simulink model "CubliMasterModel_Corner"  (R2025b)
settings: Solver=FixedStepAuto  StartTime=0.0  StopTime=10  FixedStep=0.001  RelTol=1e-3
values from neighbouring files (symbols this model uses):
  B0 = atan(-1/sqrt(2))    [CubeMasterModel_Corner.m]
  g = 9.81    [CubeMasterModel_Corner.m]
  IMU_st = 0.005    [CubeMasterModel_Corner.m]
  J_acctuator = J_rw+J_motor    (= 0.000472174)    [CubeMasterModel_Corner.m]
  K = zeros(3,8)    [CubeMasterModel_Corner.m]
  Km = 0.05    [CubeMasterModel_Corner.m]
  KV = 195    [CubeMasterModel_Corner.m]
  m = 3    [CubeMasterModel_Corner.m]
  M_battery = 100    [CubeMasterModel_Corner.m]
  M_core = 70    [CubeMasterModel_Corner.m]
  M_frame = 6*6 + 2.5*4    (= 46)    [CubeMasterModel_Corner.m]
  M_motor = 110    [CubeMasterModel_Corner.m]
  M_PCB = 106.6    [CubeMasterModel_Corner.m]
  M_wheel = 145    [CubeMasterModel_Corner.m]
  T = zeros(9)    [CubeMasterModel_Corner.m]
  Tmax = 0.25    [CubeMasterModel_Corner.m]
  TorqueRate = 0.1/0.005    (= 20)    [CubeMasterModel_Corner.m]
  Ts = 0.005    [CubeMasterModel_Corner.m]
  Y0 = pi/4    (= 0.785398163397)    [CubeMasterModel_Corner.m]
undefined symbols (not defined in the file or in its folder): X, Y, Z
libraries: sm_lib x39, nesl_utility x23, simulink x11
settings Model: Creator=Daniel  LastModifiedBy=Daniel

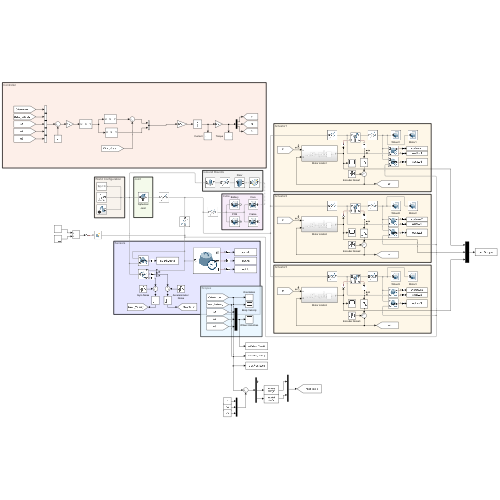
[thumbnail: Simulink's stored preview of the top-level diagram]
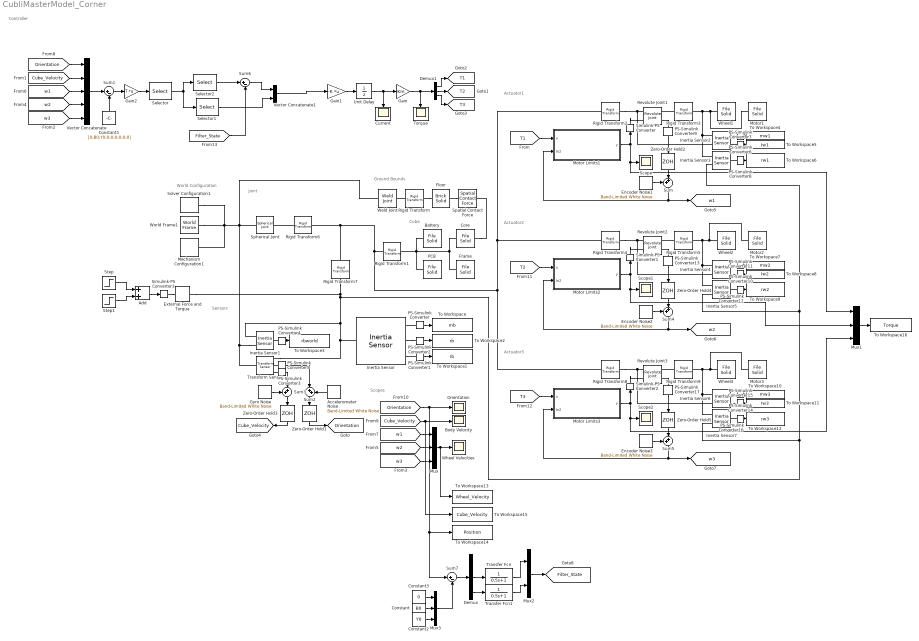
== system CubliMasterModel_Corner ==
  note: Actuator1
  note: Scopes
  note: Sensors
  note: Joint
  note: Cube
  note: Ground Bounds
  note: Controller
  note: World Configuration
  note: Actuator2
  note: Actuator3
  Accelerometer Noise : simulink/Sources/Band-Limited White Noise  Cov=IMU_acc_np  Ts=IMU_st  seed=[23341]
  Add : Sum
  Battery : sm_lib/Body Elements/File Solid  ExtGeomFileName=C:\Users\Daniel\OneDrive - University of Warwick\Documents\MATLAB\Report_Models\Edge Balance\Discretised\BatteryModel.step  UnitType=Custom  ExtGeomFileUnits=mm  StepReaderType=HEX  ExportConvexHullGeometry=on  InertiaType=CalculateFromGeometry  BasedOnType=Mass  Density=1150  DensityUnits=kg/m^3  Mass=M_battery  MassUnits=g  CenterOfMass=COM_battery  CenterOfMassUnits=mm  MomentsOfInertia=I_battery  MomentsOfInertiaUnits=g*mm^2  ProductsOfInertia=P_battery  ProductsOfInertiaUnits=g*mm^2  GraphicType=FromGeometry  MarkerShape=Sphere  MarkerSize=10  GraphicVisPropType=SimpleVisualProperties  GraphicDiffuseColor=[0 0.3 0.1]  GraphicOpacity=1  GraphicSpecularColor=[0.5 0.5 0.5 1.0]  GraphicAmbientColor=[0.15 0.15 0.15 1.0]  GraphicEmissiveColor=[0.0 0.0 0.0 1.0]  GraphicShininess=75  DoExposeReferenceFrame=on  SerializedFrames=<Frames/>
  Body Velocity : Scope
      settings: ActiveDisplayYMinimum=-1224.4716207525835  ActiveDisplayYMaximum=1175.2559397382945  DataLoggingVariableName=ScopeData2
  Constant : Constant  Value=B0
  Constant1 : Constant  Value=[0;B0;Y0;0;0;0;0;0;0]
  Constant2 : Constant  Value=Y0
  Constant3 : Constant  Value=0
  Core : sm_lib/Body Elements/File Solid  ExtGeomFileName=C:\Users\Daniel\OneDrive - University of Warwick\Documents\MATLAB\Report_Models\Edge Balance\Discretised\coreModel.3mf  UnitType=Custom  ExtGeomFileUnits=mm  StepReaderType=HEX  ExportConvexHullGeometry=on  InertiaType=PointMass  BasedOnType=Mass  Density=1150  DensityUnits=kg/m^3  Mass=M_core  MassUnits=g  CenterOfMass=COM_core  CenterOfMassUnits=mm  MomentsOfInertia=I_core  MomentsOfInertiaUnits=g*mm^2  ProductsOfInertia=P_core  ProductsOfInertiaUnits=g*mm^2  GraphicType=FromGeometry  MarkerShape=Sphere  MarkerSize=10  GraphicVisPropType=SimpleVisualProperties  GraphicDiffuseColor=[0.3 0.3 0.3]  GraphicOpacity=1  GraphicSpecularColor=[0.5 0.5 0.5 1.0]  GraphicAmbientColor=[0.15 0.15 0.15 1.0]  GraphicEmissiveColor=[0.0 0.0 0.0 1.0]  GraphicShininess=75  DoExposeReferenceFrame=on  SerializedFrames=<Frames/>
  Current : Scope
      settings: ActiveDisplayYMinimum=-5.2720631408521568  ActiveDisplayYMaximum=8.6725422679254329  DataLoggingVariableName=ScopeData3
  Demux : Demux  Outputs=3
  Demux1 : Demux  Outputs=3
  Encoder Noise1 : simulink/Sources/Band-Limited White Noise  Cov=0  Ts=0.001  seed=[23341]
  Encoder Noise2 : simulink/Sources/Band-Limited White Noise  Cov=0  Ts=0.001  seed=[23341]
  Encoder Noise3 : simulink/Sources/Band-Limited White Noise  Cov=0  Ts=0.001  seed=[23341]
  External Force and Torque : sm_lib/Forces and Torques/External Force and Torque  EnableForceX=off  EnableForceY=off  EnableForceZ=off  EnableForce=off  ForceResolutionFrame=World  EnableTorqueX=off  EnableTorqueY=on  EnableTorqueZ=off  EnableTorque=off  TorqueResolutionFrame=World
  Floor : sm_lib/Body Elements/Brick Solid  BrickDimensions=[0.4 0.4 0.1]  BrickDimensionsUnits=m  ExportEntireGeometry=on  InertiaType=CalculateFromGeometry  BasedOnType=Mass  Density=1000  DensityUnits=kg/m^3  Mass=0  MassUnits=kg  CenterOfMass=[0 0 0]  CenterOfMassUnits=m  MomentsOfInertia=[1 1 1]  MomentsOfInertiaUnits=kg*m^2  ProductsOfInertia=[0 0 0]  ProductsOfInertiaUnits=kg*m^2  GraphicType=FromGeometry  MarkerShape=Sphere  MarkerSize=10  GraphicVisPropType=SimpleVisualProperties  GraphicDiffuseColor=[0.8078 0.8078 0.8078]  GraphicOpacity=1  GraphicSpecularColor=[0.5 0.5 0.5 1.0]  GraphicAmbientColor=[0.15 0.15 0.15 1.0]  GraphicEmissiveColor=[0.0 0.0 0.0 1.0]  GraphicShininess=75  DoExposeReferenceFrame=on  SerializedFrames=<Frames/>
  Frame : sm_lib/Body Elements/File Solid  ExtGeomFileName=C:\Users\Daniel\OneDrive - University of Warwick\Documents\MATLAB\Report_Models\Edge Balance\Discretised\FrameModel.3mf  UnitType=Custom  ExtGeomFileUnits=mm  StepReaderType=HEX  ExportConvexHullGeometry=on  InertiaType=CalculateFromGeometry  BasedOnType=Mass  Density=1150  DensityUnits=kg/m^3  Mass=M_frame  MassUnits=g  CenterOfMass=COM_battery  CenterOfMassUnits=mm  MomentsOfInertia=I_battery  MomentsOfInertiaUnits=g*mm^2  ProductsOfInertia=P_battery  ProductsOfInertiaUnits=g*mm^2  GraphicType=FromGeometry  MarkerShape=Sphere  MarkerSize=10  GraphicVisPropType=SimpleVisualProperties  GraphicDiffuseColor=[0.2 0.2 0.2]  GraphicOpacity=1  GraphicSpecularColor=[0.5 0.5 0.5 1.0]  GraphicAmbientColor=[0.15 0.15 0.15 1.0]  GraphicEmissiveColor=[0.0 0.0 0.0 1.0]  GraphicShininess=75  DoExposeReferenceFrame=on  SerializedFrames=<Frames/>
  Gain : Gain  Gain=Km
  Gain1 : Gain  Gain=-K  Multiplication=Matrix(K*u)
  Gain2 : Gain  Gain=T  Multiplication=Matrix(K*u)
  Gyro Noise : simulink/Sources/Band-Limited White Noise  Cov=IMU_gyro_np  Ts=IMU_st  seed=[23341]
  Inertia Sensor : sm_lib/Body Elements/Inertia Sensor  SensorExtent=Mechanism  SpanWeldJoints=off  ExcludeGroundedBodies=off  MeasurementFrame=Attached  SenseMass=on  SenseCenterOfMass=on  SenseInertiaMatrix=on  SenseCenteredInertiaMatrix=off  SensePrincipalInertiaMatrix=off  SenseRotationMatrix=off  GraphicType=PrincipalInertiaFrame  PrincipalInertiaFrameSize=20  GraphicVisPropType=SimpleVisualProperties  GraphicDiffuseColor=[0.5 0.5 0.5]  GraphicOpacity=1  GraphicSpecularColor=[0.5 0.5 0.5 1.0]  GraphicAmbientColor=[0.15 0.15 0.15 1.0]  GraphicEmissiveColor=[0.0 0.0 0.0 1.0]  GraphicShininess=75
  Inertia Sensor1 : sm_lib/Body Elements/Inertia Sensor  SensorExtent=Mechanism  SpanWeldJoints=off  ExcludeGroundedBodies=off  MeasurementFrame=Custom  SenseMass=off  SenseCenterOfMass=on  SenseInertiaMatrix=off  SenseCenteredInertiaMatrix=off  SensePrincipalInertiaMatrix=off  SenseRotationMatrix=off  GraphicType=PrincipalInertiaFrame  PrincipalInertiaFrameSize=20  GraphicVisPropType=SimpleVisualProperties  GraphicDiffuseColor=[0.5 0.5 0.5]  GraphicOpacity=1  GraphicSpecularColor=[0.5 0.5 0.5 1.0]  GraphicAmbientColor=[0.15 0.15 0.15 1.0]  GraphicEmissiveColor=[0.0 0.0 0.0 1.0]  GraphicShininess=75
  Inertia Sensor2 : sm_lib/Body Elements/Inertia Sensor  SensorExtent=BodyGroup  SpanWeldJoints=off  ExcludeGroundedBodies=off  MeasurementFrame=Custom  SenseMass=on  SenseCenterOfMass=off  SenseInertiaMatrix=on  SenseCenteredInertiaMatrix=off  SensePrincipalInertiaMatrix=off  SenseRotationMatrix=off  GraphicType=PrincipalInertiaFrame  PrincipalInertiaFrameSize=20  GraphicVisPropType=SimpleVisualProperties  GraphicDiffuseColor=[0.5 0.5 0.5]  GraphicOpacity=1  GraphicSpecularColor=[0.5 0.5 0.5 1.0]  GraphicAmbientColor=[0.15 0.15 0.15 1.0]  GraphicEmissiveColor=[0.0 0.0 0.0 1.0]  GraphicShininess=75
  Inertia Sensor3 : sm_lib/Body Elements/Inertia Sensor  SensorExtent=BodyGroup  SpanWeldJoints=off  ExcludeGroundedBodies=off  MeasurementFrame=Custom  SenseMass=off  SenseCenterOfMass=on  SenseInertiaMatrix=off  SenseCenteredInertiaMatrix=off  SensePrincipalInertiaMatrix=off  SenseRotationMatrix=off  GraphicType=PrincipalInertiaFrame  PrincipalInertiaFrameSize=20  GraphicVisPropType=SimpleVisualProperties  GraphicDiffuseColor=[0.5 0.5 0.5]  GraphicOpacity=1  GraphicSpecularColor=[0.5 0.5 0.5 1.0]  GraphicAmbientColor=[0.15 0.15 0.15 1.0]  GraphicEmissiveColor=[0.0 0.0 0.0 1.0]  GraphicShininess=75
  Inertia Sensor4 : sm_lib/Body Elements/Inertia Sensor  SensorExtent=BodyGroup  SpanWeldJoints=off  ExcludeGroundedBodies=off  MeasurementFrame=Custom  SenseMass=on  SenseCenterOfMass=off  SenseInertiaMatrix=on  SenseCenteredInertiaMatrix=off  SensePrincipalInertiaMatrix=off  SenseRotationMatrix=off  GraphicType=PrincipalInertiaFrame  PrincipalInertiaFrameSize=20  GraphicVisPropType=SimpleVisualProperties  GraphicDiffuseColor=[0.5 0.5 0.5]  GraphicOpacity=1  GraphicSpecularColor=[0.5 0.5 0.5 1.0]  GraphicAmbientColor=[0.15 0.15 0.15 1.0]  GraphicEmissiveColor=[0.0 0.0 0.0 1.0]  GraphicShininess=75
  Inertia Sensor5 : sm_lib/Body Elements/Inertia Sensor  SensorExtent=BodyGroup  SpanWeldJoints=off  ExcludeGroundedBodies=off  MeasurementFrame=Custom  SenseMass=off  SenseCenterOfMass=on  SenseInertiaMatrix=off  SenseCenteredInertiaMatrix=off  SensePrincipalInertiaMatrix=off  SenseRotationMatrix=off  GraphicType=PrincipalInertiaFrame  PrincipalInertiaFrameSize=20  GraphicVisPropType=SimpleVisualProperties  GraphicDiffuseColor=[0.5 0.5 0.5]  GraphicOpacity=1  GraphicSpecularColor=[0.5 0.5 0.5 1.0]  GraphicAmbientColor=[0.15 0.15 0.15 1.0]  GraphicEmissiveColor=[0.0 0.0 0.0 1.0]  GraphicShininess=75
  Inertia Sensor6 : sm_lib/Body Elements/Inertia Sensor  SensorExtent=BodyGroup  SpanWeldJoints=off  ExcludeGroundedBodies=off  MeasurementFrame=Custom  SenseMass=on  SenseCenterOfMass=off  SenseInertiaMatrix=on  SenseCenteredInertiaMatrix=off  SensePrincipalInertiaMatrix=off  SenseRotationMatrix=off  GraphicType=PrincipalInertiaFrame  PrincipalInertiaFrameSize=20  GraphicVisPropType=SimpleVisualProperties  GraphicDiffuseColor=[0.5 0.5 0.5]  GraphicOpacity=1  GraphicSpecularColor=[0.5 0.5 0.5 1.0]  GraphicAmbientColor=[0.15 0.15 0.15 1.0]  GraphicEmissiveColor=[0.0 0.0 0.0 1.0]  GraphicShininess=75
  Inertia Sensor7 : sm_lib/Body Elements/Inertia Sensor  SensorExtent=BodyGroup  SpanWeldJoints=off  ExcludeGroundedBodies=off  MeasurementFrame=Custom  SenseMass=off  SenseCenterOfMass=on  SenseInertiaMatrix=off  SenseCenteredInertiaMatrix=off  SensePrincipalInertiaMatrix=off  SenseRotationMatrix=off  GraphicType=PrincipalInertiaFrame  PrincipalInertiaFrameSize=20  GraphicVisPropType=SimpleVisualProperties  GraphicDiffuseColor=[0.5 0.5 0.5]  GraphicOpacity=1  GraphicSpecularColor=[0.5 0.5 0.5 1.0]  GraphicAmbientColor=[0.15 0.15 0.15 1.0]  GraphicEmissiveColor=[0.0 0.0 0.0 1.0]  GraphicShininess=75
  Mechanism Configuration1 : sm_lib/Utilities/Mechanism Configuration  UniformGravity=Constant  GravityVector=[0 0 -9.81]  GravityVectorUnits=m/s^2  LinearizationDelta=0.001  JointModeTransitionNonlinearIterations=2
  Motor Limits1 : Subsystem
  Motor Limits2 : Subsystem
  Motor Limits3 : Subsystem
  Motor1 : sm_lib/Body Elements/File Solid  ExtGeomFileName=C:\Users\Daniel\OneDrive - University of Warwick\Documents\MATLAB\Report_Models\Edge Balance\Discretised\Motor.step  UnitType=Custom  ExtGeomFileUnits=mm  StepReaderType=HEX  ExportConvexHullGeometry=off  InertiaType=CalculateFromGeometry  BasedOnType=Mass  Density=1150  DensityUnits=kg/m^3  Mass=M_motor  MassUnits=g  CenterOfMass=[0 0 0]  CenterOfMassUnits=m  MomentsOfInertia=[0 J_acctuator 0]  MomentsOfInertiaUnits=kg*m^2  ProductsOfInertia=[0 0 0]  ProductsOfInertiaUnits=kg*m^2  GraphicType=FromGeometry  MarkerShape=Sphere  MarkerSize=10  GraphicVisPropType=SimpleVisualProperties  GraphicDiffuseColor=[0.6 0.6 0.6]  GraphicOpacity=1  GraphicSpecularColor=[0.5 0.5 0.5 1.0]  GraphicAmbientColor=[0.15 0.15 0.15 1.0]  GraphicEmissiveColor=[0.0 0.0 0.0 1.0]  GraphicShininess=75  DoExposeReferenceFrame=on  SerializedFrames=<Frames/>
  Motor2 : sm_lib/Body Elements/File Solid  ExtGeomFileName=C:\Users\Daniel\OneDrive - University of Warwick\Documents\MATLAB\Report_Models\Edge Balance\Discretised\Motor.step  UnitType=Custom  ExtGeomFileUnits=mm  StepReaderType=HEX  ExportConvexHullGeometry=off  InertiaType=CalculateFromGeometry  BasedOnType=Mass  Density=1150  DensityUnits=kg/m^3  Mass=M_motor  MassUnits=g  CenterOfMass=[0 0 0]  CenterOfMassUnits=m  MomentsOfInertia=[0 J_acctuator 0]  MomentsOfInertiaUnits=kg*m^2  ProductsOfInertia=[0 0 0]  ProductsOfInertiaUnits=kg*m^2  GraphicType=FromGeometry  MarkerShape=Sphere  MarkerSize=10  GraphicVisPropType=SimpleVisualProperties  GraphicDiffuseColor=[0.6 0.6 0.6]  GraphicOpacity=1  GraphicSpecularColor=[0.5 0.5 0.5 1.0]  GraphicAmbientColor=[0.15 0.15 0.15 1.0]  GraphicEmissiveColor=[0.0 0.0 0.0 1.0]  GraphicShininess=75  DoExposeReferenceFrame=on  SerializedFrames=<Frames/>
  Motor3 : sm_lib/Body Elements/File Solid  ExtGeomFileName=C:\Users\Daniel\OneDrive - University of Warwick\Documents\MATLAB\Report_Models\Edge Balance\Discretised\Motor.step  UnitType=Custom  ExtGeomFileUnits=mm  StepReaderType=HEX  ExportConvexHullGeometry=off  InertiaType=CalculateFromGeometry  BasedOnType=Mass  Density=1150  DensityUnits=kg/m^3  Mass=M_motor  MassUnits=g  CenterOfMass=[0 0 0]  CenterOfMassUnits=m  MomentsOfInertia=[0 J_acctuator 0]  MomentsOfInertiaUnits=kg*m^2  ProductsOfInertia=[0 0 0]  ProductsOfInertiaUnits=kg*m^2  GraphicType=FromGeometry  MarkerShape=Sphere  MarkerSize=10  GraphicVisPropType=SimpleVisualProperties  GraphicDiffuseColor=[0.6 0.6 0.6]  GraphicOpacity=1  GraphicSpecularColor=[0.5 0.5 0.5 1.0]  GraphicAmbientColor=[0.15 0.15 0.15 1.0]  GraphicEmissiveColor=[0.0 0.0 0.0 1.0]  GraphicShininess=75  DoExposeReferenceFrame=on  SerializedFrames=<Frames/>
  Mux : Mux  Inputs=3
  Mux1 : Mux  Inputs=3
  Mux2 : Mux  Inputs=2
  Mux3 : Mux  Inputs=3
  Orientation : Scope
      settings: ActiveDisplayYMinimum=-0.6735711158468275  ActiveDisplayYMaximum=1.2592628722810719
  PCB : sm_lib/Body Elements/File Solid  ExtGeomFileName=C:\Users\Daniel\OneDrive - University of Warwick\Documents\MATLAB\Report_Models\Edge Balance\Discretised\PCBModel.step  UnitType=Custom  ExtGeomFileUnits=mm  StepReaderType=HEX  ExportConvexHullGeometry=on  InertiaType=CalculateFromGeometry  BasedOnType=Mass  Density=1150  DensityUnits=kg/m^3  Mass=M_PCB  MassUnits=g  CenterOfMass=COM_battery  CenterOfMassUnits=mm  MomentsOfInertia=I_battery  MomentsOfInertiaUnits=g*mm^2  ProductsOfInertia=P_battery  ProductsOfInertiaUnits=g*mm^2  GraphicType=FromGeometry  MarkerShape=Sphere  MarkerSize=10  GraphicVisPropType=SimpleVisualProperties  GraphicDiffuseColor=[0 0.3 0.1]  GraphicOpacity=1  GraphicSpecularColor=[0.5 0.5 0.5 1.0]  GraphicAmbientColor=[0.15 0.15 0.15 1.0]  GraphicEmissiveColor=[0.0 0.0 0.0 1.0]  GraphicShininess=75  DoExposeReferenceFrame=on  SerializedFrames=<Frames/>
  PS-Simulink Converter{,1..17} (18 alike) : nesl_utility/PS-Simulink Converter  PhysicalDomain=network_engine_domain  SubClassName=ps_output  LeftPortType=input  RightPortType=output  PseudoPeriodic=off  Frequencies=[]  VectorFormat=inherit  Unit=inherit  AffineConversion=off
  Revolute Joint1 : sm_lib/Joints/Revolute Joint  JointMode=Normal  CompositeWrenchDir=FollowerOnBase  CompositeWrenchFrame=BaseFrame  SenseConstraintForce=off  SenseConstraintTorque=off  SenseTotalForce=off  SenseTotalTorque=off  PositionTargetSpecify=off  PositionTargetPriority=High  PositionTargetValue=0  PositionTargetValueUnits=deg  VelocityTargetSpecify=off  VelocityTargetPriority=High  VelocityTargetValue=0  VelocityTargetValueUnits=deg/s  EquilibriumPosition=0  EquilibriumPositionUnits=deg  SpringStiffness=0  SpringStiffnessUnits=N*m/deg  DampingCoefficient=Cw  DampingCoefficientUnits=kg*m^2/s  LowerLimitSpecify=off  LowerLimitBound=-90  LowerLimitBoundUnits=deg  LowerLimitStiffness=1e4  LowerLimitStiffnessUnits=N*m/deg  LowerLimitDamping=10  LowerLimitDampingUnits=N*m/(deg/s)  LowerLimitTransitionRegionWidth=0.1  LowerLimitTransitionRegionWidthUnits=deg  UpperLimitSpecify=off  UpperLimitBound=90  UpperLimitBoundUnits=deg  UpperLimitStiffness=1e4  UpperLimitStiffnessUnits=N*m/deg  UpperLimitDamping=10  UpperLimitDampingUnits=N*m/(deg/s)  UpperLimitTransitionRegionWidth=0.1  UpperLimitTransitionRegionWidthUnits=deg  TorqueActuationMode=InputTorque  MotionActuationMode=ComputedMotion  SensePosition=off  SenseVelocity=on  SenseAcceleration=off  SenseTorqueForce=off  SenseLowerLimitTorqueForce=off  SenseUpperLimitTorqueForce=off
  Revolute Joint2 : sm_lib/Joints/Revolute Joint  JointMode=Normal  CompositeWrenchDir=FollowerOnBase  CompositeWrenchFrame=BaseFrame  SenseConstraintForce=off  SenseConstraintTorque=off  SenseTotalForce=off  SenseTotalTorque=off  PositionTargetSpecify=off  PositionTargetPriority=High  PositionTargetValue=0  PositionTargetValueUnits=deg  VelocityTargetSpecify=off  VelocityTargetPriority=High  VelocityTargetValue=0  VelocityTargetValueUnits=deg/s  EquilibriumPosition=0  EquilibriumPositionUnits=deg  SpringStiffness=0  SpringStiffnessUnits=N*m/deg  DampingCoefficient=Cw  DampingCoefficientUnits=kg*m^2/s  LowerLimitSpecify=off  LowerLimitBound=-90  LowerLimitBoundUnits=deg  LowerLimitStiffness=1e4  LowerLimitStiffnessUnits=N*m/deg  LowerLimitDamping=10  LowerLimitDampingUnits=N*m/(deg/s)  LowerLimitTransitionRegionWidth=0.1  LowerLimitTransitionRegionWidthUnits=deg  UpperLimitSpecify=off  UpperLimitBound=90  UpperLimitBoundUnits=deg  UpperLimitStiffness=1e4  UpperLimitStiffnessUnits=N*m/deg  UpperLimitDamping=10  UpperLimitDampingUnits=N*m/(deg/s)  UpperLimitTransitionRegionWidth=0.1  UpperLimitTransitionRegionWidthUnits=deg  TorqueActuationMode=InputTorque  MotionActuationMode=ComputedMotion  SensePosition=off  SenseVelocity=on  SenseAcceleration=off  SenseTorqueForce=off  SenseLowerLimitTorqueForce=off  SenseUpperLimitTorqueForce=off
  Revolute Joint3 : sm_lib/Joints/Revolute Joint  JointMode=Normal  CompositeWrenchDir=FollowerOnBase  CompositeWrenchFrame=BaseFrame  SenseConstraintForce=off  SenseConstraintTorque=off  SenseTotalForce=off  SenseTotalTorque=off  PositionTargetSpecify=off  PositionTargetPriority=High  PositionTargetValue=0  PositionTargetValueUnits=deg  VelocityTargetSpecify=off  VelocityTargetPriority=High  VelocityTargetValue=0  VelocityTargetValueUnits=deg/s  EquilibriumPosition=0  EquilibriumPositionUnits=deg  SpringStiffness=0  SpringStiffnessUnits=N*m/deg  DampingCoefficient=Cw  DampingCoefficientUnits=kg*m^2/s  LowerLimitSpecify=off  LowerLimitBound=-90  LowerLimitBoundUnits=deg  LowerLimitStiffness=1e4  LowerLimitStiffnessUnits=N*m/deg  LowerLimitDamping=10  LowerLimitDampingUnits=N*m/(deg/s)  LowerLimitTransitionRegionWidth=0.1  LowerLimitTransitionRegionWidthUnits=deg  UpperLimitSpecify=off  UpperLimitBound=90  UpperLimitBoundUnits=deg  UpperLimitStiffness=1e4  UpperLimitStiffnessUnits=N*m/deg  UpperLimitDamping=10  UpperLimitDampingUnits=N*m/(deg/s)  UpperLimitTransitionRegionWidth=0.1  UpperLimitTransitionRegionWidthUnits=deg  TorqueActuationMode=InputTorque  MotionActuationMode=ComputedMotion  SensePosition=off  SenseVelocity=on  SenseAcceleration=off  SenseTorqueForce=off  SenseLowerLimitTorqueForce=off  SenseUpperLimitTorqueForce=off
  Rigid Transform : sm_lib/Frames and Transforms/Rigid Transform  RotationMethod=None  FollAlignAxisA=+X  BaseAlignAxisA=+Y  FollAlignAxisB=+Y  BaseAlignAxisB=+Z  RotationStandardAxis=+Z  RotationAngle=0  RotationAngleUnits=deg  RotationArbitraryAxis=[0 0 1]  RotationSequenceAxes=FollowerAxes  RotationSequence=XYX  RotationSequenceAngles=[0 0 0]  RotationSequenceAnglesUnits=deg  RotationMatrix=[1 0 0;0 1 0;0 0 1]  Quaternion=[1 0 0 0]  TranslationMethod=Cartesian  TranslationCartesianOffset=[0 0 -0.05]  TranslationCartesianOffsetUnits=m  TranslationStandardAxis=+Z  TranslationStandardOffset=0  TranslationStandardOffsetUnits=m  TranslationROffset=0  TranslationROffsetUnits=m  TranslationThetaOffset=0  TranslationThetaOffsetUnits=deg  TranslationZOffset=0  TranslationZOffsetUnits=m
  Rigid Transform1 : sm_lib/Frames and Transforms/Rigid Transform  RotationMethod=StandardAxis  FollAlignAxisA=+X  BaseAlignAxisA=+Y  FollAlignAxisB=+Y  BaseAlignAxisB=+Z  RotationStandardAxis=+Y  RotationAngle=-90  RotationAngleUnits=deg  RotationArbitraryAxis=[0 0 1]  RotationSequenceAxes=FollowerAxes  RotationSequence=XYX  RotationSequenceAngles=[35.26 45 0]  RotationSequenceAnglesUnits=deg  RotationMatrix=[1 0 0;0 1 0;0 0 1]  Quaternion=[1 0 0 0]  TranslationMethod=None  TranslationCartesianOffset=[0 0 0]  TranslationCartesianOffsetUnits=m  TranslationStandardAxis=+Z  TranslationStandardOffset=0  TranslationStandardOffsetUnits=m  TranslationROffset=0  TranslationROffsetUnits=m  TranslationThetaOffset=0  TranslationThetaOffsetUnits=deg  TranslationZOffset=0  TranslationZOffsetUnits=m
  Rigid Transform2 : sm_lib/Frames and Transforms/Rigid Transform  RotationMethod=StandardAxis  FollAlignAxisA=+X  BaseAlignAxisA=+Y  FollAlignAxisB=+Y  BaseAlignAxisB=+Z  RotationStandardAxis=+X  RotationAngle=0  RotationAngleUnits=deg  RotationArbitraryAxis=[0 0 1]  RotationSequenceAxes=FollowerAxes  RotationSequence=XYX  RotationSequenceAngles=[0 0 0]  RotationSequenceAnglesUnits=deg  RotationMatrix=[1 0 0;0 1 0;0 0 1]  Quaternion=[1 0 0 0]  TranslationMethod=Cartesian  TranslationCartesianOffset=[-0.075 0.075 0]  TranslationCartesianOffsetUnits=m  TranslationStandardAxis=+Z  TranslationStandardOffset=0  TranslationStandardOffsetUnits=m  TranslationROffset=0  TranslationROffsetUnits=m  TranslationThetaOffset=0  TranslationThetaOffsetUnits=deg  TranslationZOffset=0  TranslationZOffsetUnits=m
  Rigid Transform3 : sm_lib/Frames and Transforms/Rigid Transform  RotationMethod=StandardAxis  FollAlignAxisA=+X  BaseAlignAxisA=+Y  FollAlignAxisB=+Y  BaseAlignAxisB=+Z  RotationStandardAxis=+X  RotationAngle=90  RotationAngleUnits=deg  RotationArbitraryAxis=[0 0 1]  RotationSequenceAxes=FollowerAxes  RotationSequence=XYX  RotationSequenceAngles=[0 0 0]  RotationSequenceAnglesUnits=deg  RotationMatrix=[1 0 0;0 1 0;0 0 1]  Quaternion=[1 0 0 0]  TranslationMethod=Cartesian  TranslationCartesianOffset=[-0.075 0.075 0]  TranslationCartesianOffsetUnits=m  TranslationStandardAxis=+Z  TranslationStandardOffset=0  TranslationStandardOffsetUnits=m  TranslationROffset=0  TranslationROffsetUnits=m  TranslationThetaOffset=0  TranslationThetaOffsetUnits=deg  TranslationZOffset=0  TranslationZOffsetUnits=m
  Rigid Transform4 : sm_lib/Frames and Transforms/Rigid Transform  RotationMethod=StandardAxis  FollAlignAxisA=+X  BaseAlignAxisA=+Y  FollAlignAxisB=+Y  BaseAlignAxisB=+Z  RotationStandardAxis=+X  RotationAngle=-90  RotationAngleUnits=deg  RotationArbitraryAxis=[0 0 1]  RotationSequenceAxes=FollowerAxes  RotationSequence=XYX  RotationSequenceAngles=[0 0 0]  RotationSequenceAnglesUnits=deg  RotationMatrix=[1 0 0;0 1 0;0 0 1]  Quaternion=[1 0 0 0]  TranslationMethod=Cartesian  TranslationCartesianOffset=[-0.075 0 0.075]  TranslationCartesianOffsetUnits=m  TranslationStandardAxis=+Z  TranslationStandardOffset=0  TranslationStandardOffsetUnits=m  TranslationROffset=0  TranslationROffsetUnits=m  TranslationThetaOffset=0  TranslationThetaOffsetUnits=deg  TranslationZOffset=0  TranslationZOffsetUnits=m
  Rigid Transform5 : sm_lib/Frames and Transforms/Rigid Transform  RotationMethod=StandardAxis  FollAlignAxisA=+X  BaseAlignAxisA=+Y  FollAlignAxisB=+Y  BaseAlignAxisB=+Z  RotationStandardAxis=+X  RotationAngle=90  RotationAngleUnits=deg  RotationArbitraryAxis=[0 0 1]  RotationSequenceAxes=FollowerAxes  RotationSequence=XYX  RotationSequenceAngles=[0 0 0]  RotationSequenceAnglesUnits=deg  RotationMatrix=[1 0 0;0 1 0;0 0 1]  Quaternion=[1 0 0 0]  TranslationMethod=Cartesian  TranslationCartesianOffset=[-0.075 0.075 0]  TranslationCartesianOffsetUnits=m  TranslationStandardAxis=+Z  TranslationStandardOffset=0  TranslationStandardOffsetUnits=m  TranslationROffset=0  TranslationROffsetUnits=m  TranslationThetaOffset=0  TranslationThetaOffsetUnits=deg  TranslationZOffset=0  TranslationZOffsetUnits=m
  Rigid Transform6 : sm_lib/Frames and Transforms/Rigid Transform  RotationMethod=RotationSequence  FollAlignAxisA=+X  BaseAlignAxisA=+Y  FollAlignAxisB=+Y  BaseAlignAxisB=+Z  RotationStandardAxis=+Z  RotationAngle=0  RotationAngleUnits=deg  RotationArbitraryAxis=[0 0 1]  RotationSequenceAxes=FollowerAxes  RotationSequence=XYX  RotationSequenceAngles=[35.26 55 0]  RotationSequenceAnglesUnits=deg  RotationMatrix=[1 0 0;0 1 0;0 0 1]  Quaternion=[1 0 0 0]  TranslationMethod=None  TranslationCartesianOffset=[0 0 0]  TranslationCartesianOffsetUnits=m  TranslationStandardAxis=+Z  TranslationStandardOffset=0  TranslationStandardOffsetUnits=m  TranslationROffset=0  TranslationROffsetUnits=m  TranslationThetaOffset=0  TranslationThetaOffsetUnits=deg  TranslationZOffset=0  TranslationZOffsetUnits=m
  Rigid Transform7 : sm_lib/Frames and Transforms/Rigid Transform  RotationMethod=StandardAxis  FollAlignAxisA=+X  BaseAlignAxisA=+Y  FollAlignAxisB=+Y  BaseAlignAxisB=+Z  RotationStandardAxis=+Y  RotationAngle=-90  RotationAngleUnits=deg  RotationArbitraryAxis=[0 0 1]  RotationSequenceAxes=FollowerAxes  RotationSequence=XYX  RotationSequenceAngles=[35.26 45 0]  RotationSequenceAnglesUnits=deg  RotationMatrix=[1 0 0;0 1 0;0 0 1]  Quaternion=[1 0 0 0]  TranslationMethod=None  TranslationCartesianOffset=[0 0 0]  TranslationCartesianOffsetUnits=m  TranslationStandardAxis=+Z  TranslationStandardOffset=0  TranslationStandardOffsetUnits=m  TranslationROffset=0  TranslationROffsetUnits=m  TranslationThetaOffset=0  TranslationThetaOffsetUnits=deg  TranslationZOffset=0  TranslationZOffsetUnits=m
  Rigid Transform8 : sm_lib/Frames and Transforms/Rigid Transform  RotationMethod=StandardAxis  FollAlignAxisA=+X  BaseAlignAxisA=+Y  FollAlignAxisB=+Y  BaseAlignAxisB=+Z  RotationStandardAxis=+Y  RotationAngle=-90  RotationAngleUnits=deg  RotationArbitraryAxis=[0 0 1]  RotationSequenceAxes=FollowerAxes  RotationSequence=XYX  RotationSequenceAngles=[0 0 0]  RotationSequenceAnglesUnits=deg  RotationMatrix=[1 0 0;0 1 0;0 0 1]  Quaternion=[1 0 0 0]  TranslationMethod=Cartesian  TranslationCartesianOffset=[0 0.075 0.075]  TranslationCartesianOffsetUnits=m  TranslationStandardAxis=+Z  TranslationStandardOffset=0  TranslationStandardOffsetUnits=m  TranslationROffset=0  TranslationROffsetUnits=m  TranslationThetaOffset=0  TranslationThetaOffsetUnits=deg  TranslationZOffset=0  TranslationZOffsetUnits=m
  Rigid Transform9 : sm_lib/Frames and Transforms/Rigid Transform  RotationMethod=StandardAxis  FollAlignAxisA=+X  BaseAlignAxisA=+Y  FollAlignAxisB=+Y  BaseAlignAxisB=+Z  RotationStandardAxis=+X  RotationAngle=90  RotationAngleUnits=deg  RotationArbitraryAxis=[0 0 1]  RotationSequenceAxes=FollowerAxes  RotationSequence=XYX  RotationSequenceAngles=[0 0 0]  RotationSequenceAnglesUnits=deg  RotationMatrix=[1 0 0;0 1 0;0 0 1]  Quaternion=[1 0 0 0]  TranslationMethod=Cartesian  TranslationCartesianOffset=[-0.075 0.075 0]  TranslationCartesianOffsetUnits=m  TranslationStandardAxis=+Z  TranslationStandardOffset=0  TranslationStandardOffsetUnits=m  TranslationROffset=0  TranslationROffsetUnits=m  TranslationThetaOffset=0  TranslationThetaOffsetUnits=deg  TranslationZOffset=0  TranslationZOffsetUnits=m
  Scope : Scope
      settings: ActiveDisplayYMinimum=-1  ActiveDisplayYMaximum=1  DataLoggingVariableName=ScopeData4
  Scope1 : Scope
      settings: ActiveDisplayYMinimum=-0.21638825299854844  ActiveDisplayYMaximum=0.086796364871639109  DataLoggingVariableName=ScopeData5
  Scope2 : Scope
      settings: ActiveDisplayYMinimum=-1  ActiveDisplayYMaximum=1  DataLoggingVariableName=ScopeData6
  Selector : Selector  InputPortWidth=9  IndexOptions=Index vector (dialog)  Indices=[2:9]  OutputSizes=1
  Selector1 : Selector  InputPortWidth=8  IndexOptions=Index vector (dialog)  Indices=[3:8]  OutputSizes=1
  Selector2 : Selector  InputPortWidth=8  IndexOptions=Index vector (dialog)  Indices=[1 2]  OutputSizes=1
  Simulink-PS Converter : nesl_utility/Simulink-PS Converter  PhysicalDomain=network_engine_domain  SubClassName=ps_input  LeftPortType=input  RightPortType=output  PseudoPeriodic=off  Frequencies=[]  NoiseDistribution=none  NoiseParameters=[]  Unit=N*m  AffineConversion=off  FilteringAndDerivatives=provide  SimscapeFilterOrder=1  InputFilterTimeConstant=0.001  UdotUserProvided=0
  Simulink-PS Converter1 : nesl_utility/Simulink-PS Converter  PhysicalDomain=network_engine_domain  SubClassName=ps_input  LeftPortType=input  RightPortType=output  PseudoPeriodic=off  Frequencies=[]  NoiseDistribution=none  NoiseParameters=[]  Unit=N*m  AffineConversion=off  FilteringAndDerivatives=provide  SimscapeFilterOrder=1  InputFilterTimeConstant=0.001  UdotUserProvided=0
  Simulink-PS Converter2 : nesl_utility/Simulink-PS Converter  PhysicalDomain=network_engine_domain  SubClassName=ps_input  LeftPortType=input  RightPortType=output  PseudoPeriodic=off  Frequencies=[]  NoiseDistribution=none  NoiseParameters=[]  Unit=N*m  AffineConversion=off  FilteringAndDerivatives=provide  SimscapeFilterOrder=1  InputFilterTimeConstant=0.001  UdotUserProvided=0
  Simulink-PS Converter3 : nesl_utility/Simulink-PS Converter  PhysicalDomain=network_engine_domain  SubClassName=ps_input  LeftPortType=input  RightPortType=output  PseudoPeriodic=off  Frequencies=[]  NoiseDistribution=none  NoiseParameters=[]  Unit=1  AffineConversion=off  FilteringAndDerivatives=provide  SimscapeFilterOrder=1  InputFilterTimeConstant=0.001  UdotUserProvided=0
  Solver Configuration1 : nesl_utility/Solver Configuration  PhysicalDomain=network_engine_domain  SubClassName=solver  LeftPortType=input  RightPortType=generic  Tones=[]  Harmonics=[]  SimulateNoise=off  Profile=off  UseLocalSampling=off  EnableSwitchedLinearOptims=on  FrequencyDomain=off  UseCCode=off  RelTol=0.001  AbsTol=0.001  MinStep=1e-09  ToWorkspace=off  RevertToSquareIcSolve=off  NumHomotopyIterations=100  PhasorMode=off  PhasorModeNumHarmonics=1  ConsistencySolver=NEWTON_XTOL_AFTER_FTOL  IndexReductionMethod=DerivativeReplacement  DoDC=off  ResidualTolerance=1e-09  ConsistencyTolSource=GLOBAL  ConsistencyAbsTol=0.001  ConsistencyRelTol=0.001  ConsistencyTolFactor=0.001  UseLocalSolver=off  LocalSolverChoice=NE_BACKWARD_EULER_ADVANCER  ResolveIndetEquations=on  FunctionEvalNumThread=1  LocalSolverSampleTime=0.001  DoFixedCost=off  MaxNonlinIter=3  MaxModeIter=2  ComputeImpulses=off  ImpulseIterations=2  LinearAlgebra=auto  LinearAlgebraNumThread=0  EquationFormulation=NE_TIME_EF  DelaysMemoryBudget=1024  AutomaticFiltering=on  FilteringTimeConstant=0.001  PartitionStorageMethod=AS_NEEDED  PartitionMemoryBudget=1024  PartitionMethod=ROBUST  MultibodyUseLocalSolver=off  MultibodyLocalSolverChoice=ODE1  MultibodyLocalSolverSampleTime=0.001
  Spatial Contact Force : sm_lib/Forces and Torques/Spatial Contact Force  SenseSeparationDistance=off  NormalForceType=SmoothSpringDamper  NormalStiffness=1e5  NormalStiffnessUnits=N/m  NormalDamping=1e3  NormalDampingUnits=N/(m/s)  NormalTransitionRegionWidth=1e-4  NormalTransitionRegionWidthUnits=m  FrictionType=SmoothStickSlip  CoefficientOfStaticFriction=0.5  CoefficientOfDynamicFriction=0.3  FrictionalCriticalVelocity=1e-3  FrictionalCriticalVelocityUnits=m/s  SenseContactSignal=off  SensePenetrationDepth=off  SenseNormalVelocity=off  SenseTangentialVelocity=off  SensingForceTorqueDirection=BaseOnFollower  SensingForceTorqueResolutionFrame=ContactFrame  SenseNormalForce=off  SenseNormalForceMagnitude=off  SenseNormalTorque=off  SenseFrictionalForce=off  SenseFrictionalForceMagnitude=off  SenseFrictionalTorque=off  SenseTotalForce=off  SenseTotalTorque=off  SenseContactBaseRotation=off  SenseContactBaseTranslation=off  SenseContactFollowerRotation=off  SenseContactFollowerTranslation=off  ZeroCrossDetectContactStartAndEnd=off
  Spherical Joint : sm_lib/Joints/Spherical Joint  JointMode=Normal  CompositeWrenchDir=FollowerOnBase  CompositeWrenchFrame=BaseFrame  SenseConstraintForce=off  SenseConstraintTorque=off  SenseTotalForce=off  SenseTotalTorque=off  PositionTargetSpecify=off  PositionTargetPriority=High  PositionTargetRotationMethod=None  PositionTargetFollAlignAxisA=+X  PositionTargetBaseAlignAxisA=+Y  PositionTargetFollAlignAxisB=+Y  PositionTargetBaseAlignAxisB=+Z  PositionTargetRotationStandardAxis=+Z  PositionTargetRotationAngle=0  PositionTargetRotationAngleUnits=deg  PositionTargetRotationArbitraryAxis=[0 0 1]  PositionTargetRotationSequenceAxes=FollowerAxes  PositionTargetRotationSequence=XYX  PositionTargetRotationSequenceAngles=[0 0 0]  PositionTargetRotationSequenceAnglesUnits=deg  PositionTargetRotationMatrix=[1 0 0;0 1 0;0 0 1]  PositionTargetQuaternion=[1 0 0 0]  VelocityTargetSpecify=off  VelocityTargetPriority=High  VelocityTargetValue=[0 0 0]  VelocityTargetValueUnits=deg/s  VelocityTargetInFollowerFrame=on  EqPosRotationMethod=None  EqPosFollAlignAxisA=+X  EqPosBaseAlignAxisA=+Y  EqPosFollAlignAxisB=+Y  EqPosBaseAlignAxisB=+Z  EqPosRotationStandardAxis=+Z  EqPosRotationAngle=0  EqPosRotationAngleUnits=deg  EqPosRotationArbitraryAxis=[0 0 1]  EqPosRotationSequenceAxes=FollowerAxes  EqPosRotationSequence=XYX  EqPosRotationSequenceAngles=[0 0 0]  EqPosRotationSequenceAnglesUnits=deg  EqPosRotationMatrix=[1 0 0;0 1 0;0 0 1]  EqPosQuaternion=[1 0 0 0]  SpringStiffness=0  SpringStiffnessUnits=N*m/deg  DampingCoefficient=0  DampingCoefficientUnits=N*m/(deg/s)  LowerLimitSpecify=off  LowerLimitBound=15  LowerLimitBoundUnits=deg  LowerLimitStiffness=1e4  LowerLimitStiffnessUnits=N*m/deg  LowerLimitDamping=10  LowerLimitDampingUnits=N*m/(deg/s)  LowerLimitTransitionRegionWidth=0.1  LowerLimitTransitionRegionWidthUnits=deg  UpperLimitSpecify=off  UpperLimitBound=45  UpperLimitBoundUnits=deg  UpperLimitStiffness=1e4  UpperLimitStiffnessUnits=N*m/deg  UpperLimitDamping=10  UpperLimitDampingUnits=N*m/(deg/s)  UpperLimitTransitionRegionWidth=0.1  UpperLimitTransitionRegionWidthUnits=deg  TorqueActuationMode=NoTorque  ActuateTorqueX=off  ActuateTorqueY=off  ActuateTorqueZ=off  ActuateTorque=off  ActuationFrame=BaseFrame  SensePosition=off  SenseVelocityX=off  SenseVelocityY=off  SenseVelocityZ=off  SenseVelocity=off  SenseAccelerationX=off  SenseAccelerationY=off  SenseAccelerationZ=off  SenseAcceleration=off  SenseLowerLimitTorqueMag=off  SenseUpperLimitTorqueMag=off  SensingFrame=BaseFrame
  Step : Step  Time=5  After=0.25  SampleTime=0
  Step1 : Step  Time=5.1  After=-0.25  SampleTime=0
  Sum{,3..5} (4 alike) : Sum  Inputs=++|
  Sum1 : Sum  Inputs=|+-
  Sum2 : Sum  Inputs=|++
  Sum6 : Sum  Inputs=|+-
  Sum7 : Sum  Inputs=|+-
  To Workspace : ToWorkspace  VariableName=mb  SampleTime=-1
  To Workspace1 : ToWorkspace  VariableName=Ib  SampleTime=-1
  To Workspace10 : ToWorkspace  VariableName=mw3  SampleTime=-1
  To Workspace11 : ToWorkspace  VariableName=Iw3  SampleTime=-1
  To Workspace12 : ToWorkspace  VariableName=rw3  SampleTime=-1
  To Workspace13 : ToWorkspace  VariableName=Wheel_Velocity  SaveFormat=Timeseries  SampleTime=-1
  To Workspace14 : ToWorkspace  VariableName=Position  SaveFormat=Timeseries  SampleTime=-1
  To Workspace15 : ToWorkspace  VariableName=Cube_Velocity  SaveFormat=Timeseries  SampleTime=-1
  To Workspace16 : ToWorkspace  VariableName=Torque  SaveFormat=Timeseries  SampleTime=-1
  To Workspace2 : ToWorkspace  VariableName=rb  SampleTime=-1
  To Workspace3 : ToWorkspace  VariableName=rbworld  SampleTime=-1
  To Workspace4 : ToWorkspace  VariableName=mw1  SampleTime=-1
  To Workspace5 : ToWorkspace  VariableName=Iw1  SampleTime=-1
  To Workspace6 : ToWorkspace  VariableName=rw1  SampleTime=-1
  To Workspace7 : ToWorkspace  VariableName=mw2  SampleTime=-1
  To Workspace8 : ToWorkspace  VariableName=Iw2  SampleTime=-1
  To Workspace9 : ToWorkspace  VariableName=rw2  SampleTime=-1
  Torque : Scope
      settings: ActiveDisplayYMinimum=-0.26360315704260784  ActiveDisplayYMaximum=0.43362711339627164  DataLoggingVariableName=ScopeData8
  Transfer Fcn : TransferFcn  Denominator=[0.5 1]
  Transfer Fcn1 : TransferFcn  Denominator=[0.5 1]
  Transform Sensor : sm_lib/Frames and Transforms/Transform Sensor  MeasurementFrame=World  RotationSequence=ZYX  SenseAngle=off  SenseAxis=off  SenseQ=off  SenseR=off  SenseRotationSequence=on  SenseOmegaX=off  SenseOmegaY=off  SenseOmegaZ=off  SenseOmega=on  SenseQDot=off  SenseRDot=off  SenseRotationSequenceDot=off  SenseAlphaX=off  SenseAlphaY=off  SenseAlphaZ=off  SenseAlpha=off  SenseQDDot=off  SenseRDDot=off  SenseX=off  SenseY=off  SenseZ=off  SenseXYZ=off  SenseRad=off  SenseAzim=off  SenseDist=off  SenseInc=off  SenseXDot=off  SenseYDot=off  SenseZDot=off  SenseXYZDot=off  SenseRadDot=off  SenseAzimDot=off  SenseDistDot=off  SenseIncDot=off  SenseXDDot=off  SenseYDDot=off  SenseZDDot=off  SenseXYZDDot=off  SenseRadDDot=off  SenseAzimDDot=off  SenseDistDDot=off  SenseIncDDot=off
  Unit Delay : UnitDelay  SampleTime=Ts  HasFrameUpgradeWarning=on
  Vector Concatenate : Concatenate  NumInputs=5
  Vector Concatenate1 : Concatenate
  Weld Joint : sm_lib/Joints/Weld Joint  JointMode=Normal  CompositeWrenchDir=FollowerOnBase  CompositeWrenchFrame=BaseFrame  SenseConstraintForce=off  SenseConstraintTorque=off  SenseTotalForce=off  SenseTotalTorque=off
  Wheel Velocities : Scope
      settings: ActiveDisplayYMinimum=-81.869932207792615  ActiveDisplayYMaximum=92.501267841801237
  Wheel1 : sm_lib/Body Elements/File Solid  ExtGeomFileName=C:\Users\Daniel\OneDrive - University of Warwick\Documents\MATLAB\Report_Models\Edge Balance\Discretised\RW.step  UnitType=Custom  ExtGeomFileUnits=mm  StepReaderType=HEX  ExportConvexHullGeometry=off  InertiaType=CalculateFromGeometry  BasedOnType=Mass  Density=1150  DensityUnits=kg/m^3  Mass=M_wheel  MassUnits=g  CenterOfMass=[0 0 0]  CenterOfMassUnits=m  MomentsOfInertia=[0 J_acctuator 0]  MomentsOfInertiaUnits=kg*m^2  ProductsOfInertia=[0 0 0]  ProductsOfInertiaUnits=kg*m^2  GraphicType=FromGeometry  MarkerShape=Sphere  MarkerSize=10  GraphicVisPropType=SimpleVisualProperties  GraphicDiffuseColor=[0.77 0.55 0]  GraphicOpacity=1  GraphicSpecularColor=[0.5 0.5 0.5 1.0]  GraphicAmbientColor=[0.15 0.15 0.15 1.0]  GraphicEmissiveColor=[0.0 0.0 0.0 1.0]  GraphicShininess=75  DoExposeReferenceFrame=on  SerializedFrames=<Frames/>
  Wheel2 : sm_lib/Body Elements/File Solid  ExtGeomFileName=C:\Users\Daniel\OneDrive - University of Warwick\Documents\MATLAB\Report_Models\Edge Balance\Discretised\RW.step  UnitType=Custom  ExtGeomFileUnits=mm  StepReaderType=HEX  ExportConvexHullGeometry=off  InertiaType=CalculateFromGeometry  BasedOnType=Mass  Density=1150  DensityUnits=kg/m^3  Mass=M_wheel  MassUnits=g  CenterOfMass=[0 0 0]  CenterOfMassUnits=m  MomentsOfInertia=[0 J_acctuator 0]  MomentsOfInertiaUnits=kg*m^2  ProductsOfInertia=[0 0 0]  ProductsOfInertiaUnits=kg*m^2  GraphicType=FromGeometry  MarkerShape=Sphere  MarkerSize=10  GraphicVisPropType=SimpleVisualProperties  GraphicDiffuseColor=[0.77 0.55 0]  GraphicOpacity=1  GraphicSpecularColor=[0.5 0.5 0.5 1.0]  GraphicAmbientColor=[0.15 0.15 0.15 1.0]  GraphicEmissiveColor=[0.0 0.0 0.0 1.0]  GraphicShininess=75  DoExposeReferenceFrame=on  SerializedFrames=<Frames/>
  Wheel3 : sm_lib/Body Elements/File Solid  ExtGeomFileName=C:\Users\Daniel\OneDrive - University of Warwick\Documents\MATLAB\Report_Models\Edge Balance\Discretised\RW.step  UnitType=Custom  ExtGeomFileUnits=mm  StepReaderType=HEX  ExportConvexHullGeometry=off  InertiaType=CalculateFromGeometry  BasedOnType=Mass  Density=1150  DensityUnits=kg/m^3  Mass=M_wheel  MassUnits=g  CenterOfMass=[0 0 0]  CenterOfMassUnits=m  MomentsOfInertia=[0 J_acctuator 0]  MomentsOfInertiaUnits=kg*m^2  ProductsOfInertia=[0 0 0]  ProductsOfInertiaUnits=kg*m^2  GraphicType=FromGeometry  MarkerShape=Sphere  MarkerSize=10  GraphicVisPropType=SimpleVisualProperties  GraphicDiffuseColor=[0.77 0.55 0]  GraphicOpacity=1  GraphicSpecularColor=[0.5 0.5 0.5 1.0]  GraphicAmbientColor=[0.15 0.15 0.15 1.0]  GraphicEmissiveColor=[0.0 0.0 0.0 1.0]  GraphicShininess=75  DoExposeReferenceFrame=on  SerializedFrames=<Frames/>
  World Frame1 : sm_lib/Frames and Transforms/World Frame
  Zero-Order Hold{1..5} (5 alike) : ZeroOrderHold  SampleTime=Ts
  tag scope: Cube_Velocity=global, Filter_State=global, Orientation=global, T1=global, T2=global, T3=global, w1=global, w2=global, w3=global
  wires:
  Unit Delay/1 -> Current/1, Gain/1
  Gain/1 -> Demux1/1, Torque/1
  Demux1/3 -> [T3]
  Demux1/2 -> [T2]
  Demux1/1 -> [T1]
  Gain2/1 -> Selector/1
  Mux/1 -> Wheel Velocities/1, To Workspace13/1
  [w3] -> Vector Concatenate/5
  [w1] -> Vector Concatenate/3
  [w2] -> Vector Concatenate/4
  Sum1/1 -> Gain2/1
  Vector Concatenate/1 -> Sum1/1
  Constant1/1 -> Sum1/2
  [Cube_Velocity] -> Vector Concatenate/2
  Gain1/1 -> Unit Delay/1
  [w1] -> Mux/1
  [w2] -> Mux/2
  [w3] -> Mux/3
  [Orientation] -> Orientation/1, Sum7/1, To Workspace14/1
  [Cube_Velocity] -> To Workspace15/1, Body Velocity/1
  PS-Simulink Converter/1 -> To Workspace/1
  PS-Simulink Converter1/1 -> To Workspace1/1
  PS-Simulink Converter2/1 -> To Workspace2/1
  Zero-Order Hold3/1 -> [Cube_Velocity]
  Zero-Order Hold1/1 -> [Orientation]
  PS-Simulink Converter4/1 -> To Workspace3/1
  PS-Simulink Converter3/1 -> Sum3/2
  Sum2/1 -> Zero-Order Hold1/1
  Sum3/1 -> Zero-Order Hold3/1
  Gyro Noise/1 -> Sum3/1
  Accelerometer Noise/1 -> Sum2/2
  PS-Simulink Converter5/1 -> Sum2/1
  Sum/1 -> [w1], Motor Limits1/2(In2)
  Zero-Order Hold2/1 -> Sum/2
  Encoder Noise1/1 -> Sum/1
  Motor Limits1/1(y) -> Simulink-PS Converter/1, Mux1/1, Scope/1
  [T1] -> Motor Limits1/1(u)
  PS-Simulink Converter9/1 -> Zero-Order Hold2/1
  PS-Simulink Converter8/1 -> To Workspace6/1
  PS-Simulink Converter7/1 -> To Workspace5/1
  PS-Simulink Converter6/1 -> To Workspace4/1
  [T2] -> Motor Limits2/1(u)
  PS-Simulink Converter13/1 -> Zero-Order Hold4/1
  Motor Limits2/1(y) -> Mux1/2, Scope1/1, Simulink-PS Converter1/1
  Zero-Order Hold4/1 -> Sum4/2
  Encoder Noise2/1 -> Sum4/1
  Sum4/1 -> [w2], Motor Limits2/2(In2)
  PS-Simulink Converter10/1 -> To Workspace7/1
  PS-Simulink Converter12/1 -> To Workspace9/1
  PS-Simulink Converter11/1 -> To Workspace8/1
  [T3] -> Motor Limits3/1(u)
  PS-Simulink Converter17/1 -> Zero-Order Hold5/1
  Motor Limits3/1(y) -> Simulink-PS Converter2/1, Mux1/3, Scope2/1
  Zero-Order Hold5/1 -> Sum5/2
  Encoder Noise3/1 -> Sum5/1
  Sum5/1 -> [w3], Motor Limits3/2(In2)
  PS-Simulink Converter14/1 -> To Workspace10/1
  PS-Simulink Converter16/1 -> To Workspace12/1
  PS-Simulink Converter15/1 -> To Workspace11/1
  Add/1 -> Simulink-PS Converter3/1
  Step/1 -> Add/1
  Step1/1 -> Add/2
  Mux1/1 -> To Workspace16/1
  [Orientation] -> Vector Concatenate/1
  Mux2/1 -> [Filter_State]
  Demux/2 -> Transfer Fcn/1
  Demux/3 -> Transfer Fcn1/1
  Selector2/1 -> Sum6/1
  Vector Concatenate1/1 -> Gain1/1
  Selector1/1 -> Vector Concatenate1/2
  [Filter_State] -> Sum6/2
  Sum6/1 -> Vector Concatenate1/1
  Selector/1 -> Selector2/1, Selector1/1
  Transfer Fcn/1 -> Mux2/1
  Transfer Fcn1/1 -> Mux2/2
  Sum7/1 -> Demux/1
  Mux3/1 -> Sum7/2
  Constant2/1 -> Mux3/3
  Constant3/1 -> Mux3/1
  Constant/1 -> Mux3/2
  connections:
  Rigid Transform/LConn1 -- Weld Joint/RConn1
  Rigid Transform/RConn1 -- Floor/RConn1
  Floor/LConn1 -- Spatial Contact Force/LConn1
  Rigid Transform8/LConn1 -- Rigid Transform4/LConn1 -- Rigid Transform2/LConn1 -- Rigid Transform1/LConn1 -- Rigid Transform6/RConn1 -- Rigid Transform7/LConn1
  Rigid Transform6/LConn1 -- Spherical Joint/RConn1
  Core/LConn1 -- Spatial Contact Force/RConn1
  PS-Simulink Converter1/LConn1 -- Inertia Sensor/RConn3
  Inertia Sensor/RConn2 -- PS-Simulink Converter2/LConn1
  PS-Simulink Converter/LConn1 -- Inertia Sensor/RConn1
  Transform Sensor/RConn3 -- PS-Simulink Converter3/LConn1
  PS-Simulink Converter5/LConn1 -- Transform Sensor/RConn2
  Inertia Sensor1/RConn1 -- PS-Simulink Converter4/LConn1
  Inertia Sensor2/LConn1 -- Inertia Sensor3/LConn1 -- Motor1/RConn1 -- Wheel1/RConn1 -- Rigid Transform3/RConn1
  PCB/RConn1 -- Rigid Transform1/RConn1 -- Battery/RConn1 -- Frame/RConn1 -- Core/RConn1
  Revolute Joint1/RConn2 -- PS-Simulink Converter9/LConn1
  Transform Sensor/RConn1 -- External Force and Torque/RConn1 -- Rigid Transform7/RConn1 -- Inertia Sensor7/LConn2 -- Inertia Sensor5/LConn2 -- Inertia Sensor3/LConn2 -- Inertia Sensor1/LConn1 -- Inertia Sensor/LConn1
  PS-Simulink Converter8/LConn1 -- Inertia Sensor3/RConn1
  Inertia Sensor2/RConn2 -- PS-Simulink Converter7/LConn1
  Inertia Sensor2/RConn1 -- PS-Simulink Converter6/LConn1
  Simulink-PS Converter/RConn1 -- Revolute Joint1/LConn2
  Rigid Transform3/LConn1 -- Revolute Joint1/RConn1
  Rigid Transform2/RConn1 -- Inertia Sensor2/LConn2 -- Revolute Joint1/LConn1
  Inertia Sensor4/LConn1 -- Inertia Sensor5/LConn1 -- Motor2/RConn1 -- Wheel2/RConn1 -- Rigid Transform5/RConn1
  Revolute Joint2/LConn1 -- Rigid Transform4/RConn1 -- Inertia Sensor4/LConn2
  Inertia Sensor4/RConn2 -- PS-Simulink Converter11/LConn1
  Revolute Joint2/RConn2 -- PS-Simulink Converter13/LConn1
  PS-Simulink Converter12/LConn1 -- Inertia Sensor5/RConn1
  Inertia Sensor4/RConn1 -- PS-Simulink Converter10/LConn1
  Simulink-PS Converter1/RConn1 -- Revolute Joint2/LConn2
  Rigid Transform5/LConn1 -- Revolute Joint2/RConn1
  Inertia Sensor6/LConn1 -- Inertia Sensor7/LConn1 -- Motor3/RConn1 -- Wheel3/RConn1 -- Rigid Transform9/RConn1
  Revolute Joint3/LConn1 -- Rigid Transform8/RConn1 -- Inertia Sensor6/LConn2
  Inertia Sensor6/RConn2 -- PS-Simulink Converter15/LConn1
  Revolute Joint3/RConn2 -- PS-Simulink Converter17/LConn1
  PS-Simulink Converter16/LConn1 -- Inertia Sensor7/RConn1
  Inertia Sensor6/RConn1 -- PS-Simulink Converter14/LConn1
  Simulink-PS Converter2/RConn1 -- Revolute Joint3/LConn2
  Rigid Transform9/LConn1 -- Revolute Joint3/RConn1
  Inertia Sensor1/LConn2 -- World Frame1/RConn1 -- Mechanism Configuration1/RConn1 -- Solver Configuration1/RConn1 -- Weld Joint/LConn1 -- Spherical Joint/LConn1 -- Transform Sensor/LConn1
  Simulink-PS Converter3/RConn1 -- External Force and Torque/LConn1

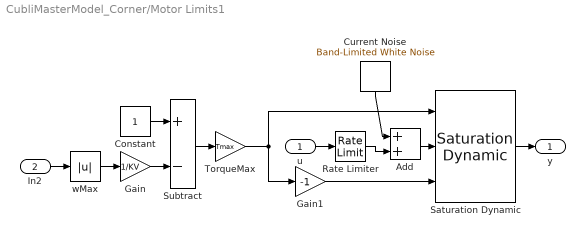
== system CubliMasterModel_Corner/Motor Limits1 ==
  u : Inport
  In2 : Inport  Port=2
  Add : Sum
  Constant : Constant
  Current Noise : simulink/Sources/Band-Limited White Noise  Cov=0  Ts=0.001  seed=[23341]
  Gain : Gain  Gain=1/KV
  Gain1 : Gain  Gain=-1
  Rate Limiter : RateLimiter  RisingSlewLimit=TorqueRate  FallingSlewLimit=-TorqueRate  SampleTimeMode=inherited
  Saturation Dynamic : simulink/Discontinuities/Saturation Dynamic  OutMin=[]  OutMax=[]  OutDataTypeStr=Inherit: Same as second input  OutDataType=fixdt(1, 16)  OutScaling=2^-10  DoSatur=off
  Subtract : Sum  Inputs=+-
  TorqueMax : Gain  Gain=Tmax
  wMax : Abs  SaturateOnIntegerOverflow=off
  y : Outport
  wires:
  In2/1 -> wMax/1
  Constant/1 -> Subtract/1
  wMax/1 -> Gain/1
  TorqueMax/1 -> Gain1/1, Saturation Dynamic/1
  u/1 -> Rate Limiter/1
  Gain1/1 -> Saturation Dynamic/3
  Gain/1 -> Subtract/2
  Subtract/1 -> TorqueMax/1
  Saturation Dynamic/1 -> y/1
  Rate Limiter/1 -> Add/2
  Add/1 -> Saturation Dynamic/2
  Current Noise/1 -> Add/1

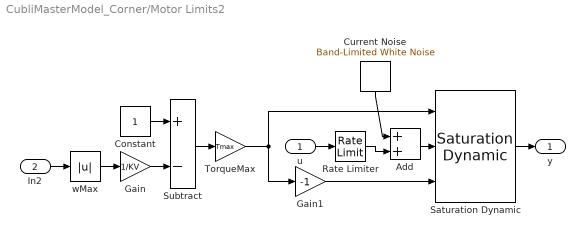
== system CubliMasterModel_Corner/Motor Limits2 ==
  u : Inport
  In2 : Inport  Port=2
  Add : Sum
  Constant : Constant
  Current Noise : simulink/Sources/Band-Limited White Noise  Cov=0  Ts=0.001  seed=[23341]
  Gain : Gain  Gain=1/KV
  Gain1 : Gain  Gain=-1
  Rate Limiter : RateLimiter  RisingSlewLimit=TorqueRate  FallingSlewLimit=-TorqueRate  SampleTimeMode=inherited
  Saturation Dynamic : simulink/Discontinuities/Saturation Dynamic  OutMin=[]  OutMax=[]  OutDataTypeStr=Inherit: Same as second input  OutDataType=fixdt(1, 16)  OutScaling=2^-10  DoSatur=off
  Subtract : Sum  Inputs=+-
  TorqueMax : Gain  Gain=Tmax
  wMax : Abs  SaturateOnIntegerOverflow=off
  y : Outport
  wires:
  In2/1 -> wMax/1
  Constant/1 -> Subtract/1
  wMax/1 -> Gain/1
  TorqueMax/1 -> Gain1/1, Saturation Dynamic/1
  u/1 -> Rate Limiter/1
  Gain1/1 -> Saturation Dynamic/3
  Gain/1 -> Subtract/2
  Subtract/1 -> TorqueMax/1
  Saturation Dynamic/1 -> y/1
  Rate Limiter/1 -> Add/2
  Add/1 -> Saturation Dynamic/2
  Current Noise/1 -> Add/1

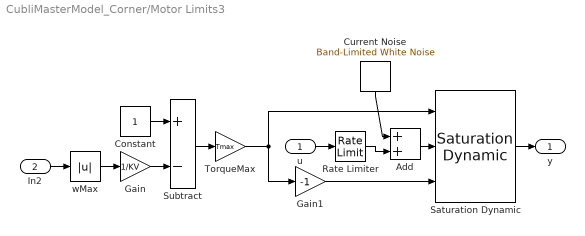
== system CubliMasterModel_Corner/Motor Limits3 ==
  u : Inport
  In2 : Inport  Port=2
  Add : Sum
  Constant : Constant
  Current Noise : simulink/Sources/Band-Limited White Noise  Cov=0  Ts=0.001  seed=[23341]
  Gain : Gain  Gain=1/KV
  Gain1 : Gain  Gain=-1
  Rate Limiter : RateLimiter  RisingSlewLimit=TorqueRate  FallingSlewLimit=-TorqueRate  SampleTimeMode=inherited
  Saturation Dynamic : simulink/Discontinuities/Saturation Dynamic  OutMin=[]  OutMax=[]  OutDataTypeStr=Inherit: Same as second input  OutDataType=fixdt(1, 16)  OutScaling=2^-10  DoSatur=off
  Subtract : Sum  Inputs=+-
  TorqueMax : Gain  Gain=Tmax
  wMax : Abs  SaturateOnIntegerOverflow=off
  y : Outport
  wires:
  In2/1 -> wMax/1
  Constant/1 -> Subtract/1
  wMax/1 -> Gain/1
  TorqueMax/1 -> Gain1/1, Saturation Dynamic/1
  u/1 -> Rate Limiter/1
  Gain1/1 -> Saturation Dynamic/3
  Gain/1 -> Subtract/2
  Subtract/1 -> TorqueMax/1
  Saturation Dynamic/1 -> y/1
  Rate Limiter/1 -> Add/2
  Add/1 -> Saturation Dynamic/2
  Current Noise/1 -> Add/1
